simulink model "MANUFACTURINGCELL"  (R2026a)
settings: Solver=VariableStepAuto  StopTime=1000.0
undefined symbols (not defined in the file): m, n
libraries: sldelib x3
settings Model: Creator=Sayandip Mallick  LastModifiedBy=Nilesh Banik

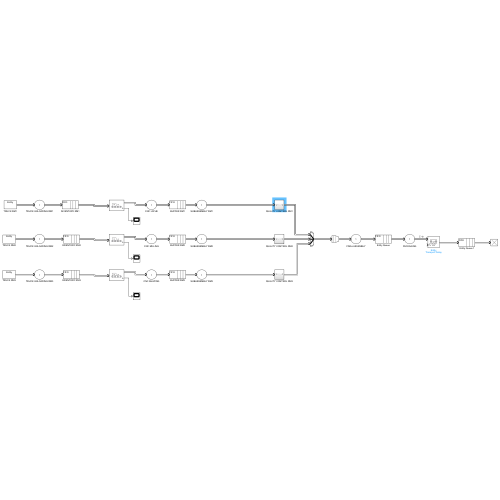
[thumbnail: Simulink's stored preview of the top-level diagram]
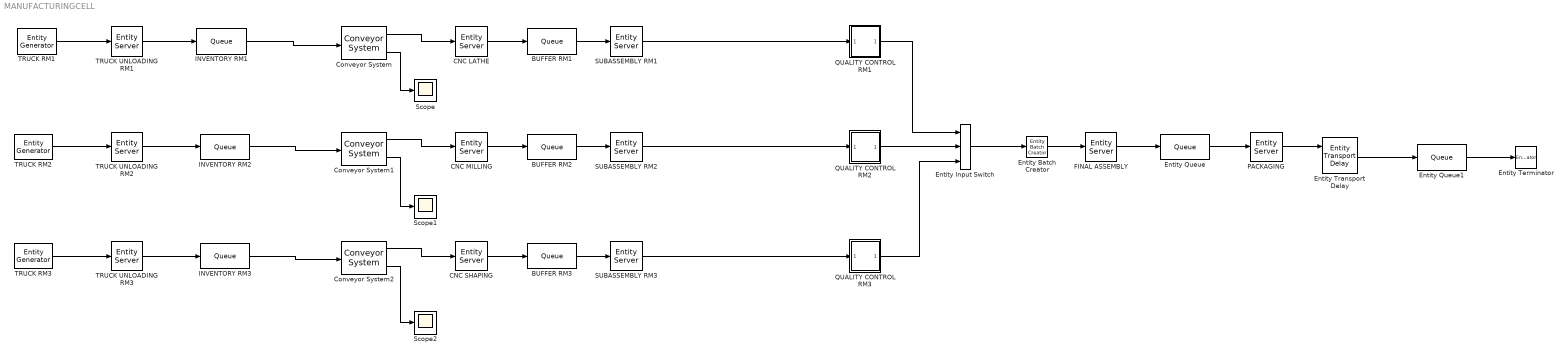
== system MANUFACTURINGCELL ==
  BUFFER RM1 : Queue  InputPortMessageModes=m  OutputPortMessageModes=m
  BUFFER RM2 : Queue  InputPortMessageModes=m  OutputPortMessageModes=m
  BUFFER RM3 : Queue  InputPortMessageModes=m  OutputPortMessageModes=m
  CNC LATHE : EntityServer  InputPortMessageModes=m  OutputPortMessageModes=m  Capacity=1
  CNC MILLING : EntityServer  InputPortMessageModes=m  OutputPortMessageModes=m  Capacity=1
  CNC SHAPING : EntityServer  InputPortMessageModes=m  OutputPortMessageModes=m  Capacity=1
  Conveyor System : sldelib/Conveyor System  mConveyorLength=10  mConveyorSpeedSource=Dialog  mConveyorSpeed=2  mInitialConveyorSpeed=1000  mMinDisBetEntity=1  mEntityLengthSource=Dialog  mEntityLength=1  mEntityLengthAttrName=Length  mOutputBlockedOpt=Pause  mErrorUponFullOpt=on  mNumEntitiesDepOpt=off  mNumEntitiesInBlockOpt=on  mEntityPendingOpt=off  mNumExtractedFromBlockOpt=off  mConveyorSpeedOpt=off
  Conveyor System1 : sldelib/Conveyor System  mConveyorLength=10  mConveyorSpeedSource=Dialog  mConveyorSpeed=2  mInitialConveyorSpeed=1000  mMinDisBetEntity=1  mEntityLengthSource=Dialog  mEntityLength=1  mEntityLengthAttrName=Length  mOutputBlockedOpt=Pause  mErrorUponFullOpt=on  mNumEntitiesDepOpt=off  mNumEntitiesInBlockOpt=on  mEntityPendingOpt=off  mNumExtractedFromBlockOpt=off  mConveyorSpeedOpt=off
  Conveyor System2 : sldelib/Conveyor System  mConveyorLength=10  mConveyorSpeedSource=Dialog  mConveyorSpeed=2  mInitialConveyorSpeed=1000  mMinDisBetEntity=1  mEntityLengthSource=Dialog  mEntityLength=1  mEntityLengthAttrName=Length  mOutputBlockedOpt=Pause  mErrorUponFullOpt=on  mNumEntitiesDepOpt=off  mNumEntitiesInBlockOpt=on  mEntityPendingOpt=off  mNumExtractedFromBlockOpt=off  mConveyorSpeedOpt=off
  Entity Input Switch : EntityInputSwitch  InputPortMessageModes=m,m,m  OutputPortMessageModes=m  NumberInputPorts=3
      settings: InputPortMap=u1,u2,u3
  Entity Transport Delay : EntityTransportDelay  InputPortMessageModes=m,n  OutputPortMessageModes=m
  Entity Batch Creator : EntityBatchCreator  InputPortMessageModes=m  OutputPortMessageModes=m  NumberOfEntitiesInBatch=3
      settings: OutputPortMap=o4
  Entity Queue : Queue  InputPortMessageModes=m  OutputPortMessageModes=m
  Entity Queue1 : Queue  InputPortMessageModes=m  OutputPortMessageModes=m
  Entity Terminator : EntityTerminator  InputPortMessageModes=m
  FINAL ASSEMBLY : EntityServer  InputPortMessageModes=m  OutputPortMessageModes=m  Capacity=1
  INVENTORY RM1 : Queue  InputPortMessageModes=m  OutputPortMessageModes=m
  INVENTORY RM2 : Queue  InputPortMessageModes=m  OutputPortMessageModes=m
  INVENTORY RM3 : Queue  InputPortMessageModes=m  OutputPortMessageModes=m
  PACKAGING : EntityServer  InputPortMessageModes=m  OutputPortMessageModes=m  Capacity=1
  QUALITY CONTROL RM1 : Subsystem
  QUALITY CONTROL RM2 : Subsystem
  QUALITY CONTROL RM3 : Subsystem
  SUBASSEMBLY RM1 : EntityServer  InputPortMessageModes=m  OutputPortMessageModes=m  Capacity=1
  SUBASSEMBLY RM2 : EntityServer  InputPortMessageModes=m  OutputPortMessageModes=m  Capacity=1
  SUBASSEMBLY RM3 : EntityServer  InputPortMessageModes=m  OutputPortMessageModes=m  Capacity=1
  Scope : Scope
      settings: ActiveDisplayYMinimum=-0.028729918999930576  ActiveDisplayYMaximum=0.73866164792601829
  Scope1 : Scope
  Scope2 : Scope
      settings: DataLoggingVariableName=ScopeData2
  TRUCK RM1 : EntityGenerator  OutputPortMessageModes=m  Period=300  EntityType=Structured  EntityTypeName=Entity
  TRUCK RM2 : EntityGenerator  OutputPortMessageModes=m  Period=300  EntityType=Structured  EntityTypeName=Entity
  TRUCK RM3 : EntityGenerator  OutputPortMessageModes=m  Period=300  EntityType=Structured  EntityTypeName=Entity
  TRUCK UNLOADING RM1 : EntityServer  InputPortMessageModes=m  OutputPortMessageModes=m  Capacity=1
  TRUCK UNLOADING RM2 : EntityServer  InputPortMessageModes=m  OutputPortMessageModes=m  Capacity=1
  TRUCK UNLOADING RM3 : EntityServer  InputPortMessageModes=m  OutputPortMessageModes=m  Capacity=1
  wires:
  TRUCK RM1/1 -> TRUCK UNLOADING RM1/1
  TRUCK UNLOADING RM1/1 -> INVENTORY RM1/1
  INVENTORY RM1/1 -> Conveyor System/1
  TRUCK UNLOADING RM2/1 -> INVENTORY RM2/1
  TRUCK RM2/1 -> TRUCK UNLOADING RM2/1
  TRUCK UNLOADING RM3/1 -> INVENTORY RM3/1
  TRUCK RM3/1 -> TRUCK UNLOADING RM3/1
  CNC LATHE/1 -> BUFFER RM1/1
  CNC MILLING/1 -> BUFFER RM2/1
  CNC SHAPING/1 -> BUFFER RM3/1
  BUFFER RM1/1 -> SUBASSEMBLY RM1/1
  BUFFER RM2/1 -> SUBASSEMBLY RM2/1
  BUFFER RM3/1 -> SUBASSEMBLY RM3/1
  SUBASSEMBLY RM1/1 -> QUALITY CONTROL RM1/1(In1)
  SUBASSEMBLY RM2/1 -> QUALITY CONTROL RM2/1(In1)
  SUBASSEMBLY RM3/1 -> QUALITY CONTROL RM3/1(In1)
  QUALITY CONTROL RM1/1(Out1) -> Entity Input Switch/1
  QUALITY CONTROL RM2/1(Out1) -> Entity Input Switch/2
  QUALITY CONTROL RM3/1(Out1) -> Entity Input Switch/3
  Entity Input Switch/1 -> Entity Batch Creator/1
  Entity Batch Creator/1 -> FINAL ASSEMBLY/1
  FINAL ASSEMBLY/1 -> Entity Queue/1
  Entity Queue/1 -> PACKAGING/1
  PACKAGING/1 -> Entity Transport Delay/1
  Entity Transport Delay/1 -> Entity Queue1/1
  Entity Queue1/1 -> Entity Terminator/1
  Conveyor System/1 -> CNC LATHE/1
  INVENTORY RM2/1 -> Conveyor System1/1
  Conveyor System1/1 -> CNC MILLING/1
  Conveyor System2/1 -> CNC SHAPING/1
  INVENTORY RM3/1 -> Conveyor System2/1
  Conveyor System/2 -> Scope/1
  Conveyor System1/2 -> Scope1/1
  Conveyor System2/2 -> Scope2/1

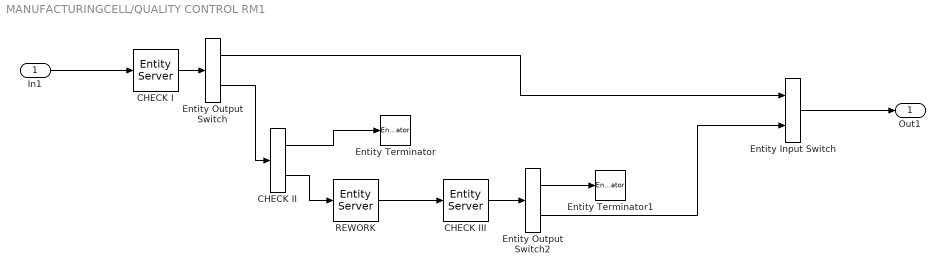
== system MANUFACTURINGCELL/QUALITY CONTROL RM1 ==
  In1 : Inport
  CHECK I : EntityServer  InputPortMessageModes=m  OutputPortMessageModes=m  Capacity=1
  CHECK II : EntityOutputSwitch  InputPortMessageModes=m  OutputPortMessageModes=m,m  SwitchAttributeName=Attribute1
  CHECK III : EntityServer  InputPortMessageModes=m  OutputPortMessageModes=m  Capacity=1
  Entity Input Switch : EntityInputSwitch  InputPortMessageModes=m,m  OutputPortMessageModes=m
  Entity Output Switch : EntityOutputSwitch  InputPortMessageModes=m  OutputPortMessageModes=m,m  SwitchingCriterion=From attribute  SwitchAttributeName=Attribute1
  Entity Output Switch2 : EntityOutputSwitch  InputPortMessageModes=m  OutputPortMessageModes=m,m  SwitchAttributeName=Attribute1
  Entity Terminator : EntityTerminator  InputPortMessageModes=m
  Entity Terminator1 : EntityTerminator  InputPortMessageModes=m
  REWORK : EntityServer  InputPortMessageModes=m  OutputPortMessageModes=m  Capacity=1
  Out1 : Outport
  wires:
  Entity Output Switch/2 -> CHECK II/1
  CHECK II/2 -> REWORK/1
  CHECK III/1 -> Entity Output Switch2/1
  Entity Output Switch2/1 -> Entity Terminator1/1
  CHECK I/1 -> Entity Output Switch/1
  REWORK/1 -> CHECK III/1
  CHECK II/1 -> Entity Terminator/1
  In1/1 -> CHECK I/1
  Entity Output Switch/1 -> Entity Input Switch/1
  Entity Output Switch2/2 -> Entity Input Switch/2
  Entity Input Switch/1 -> Out1/1

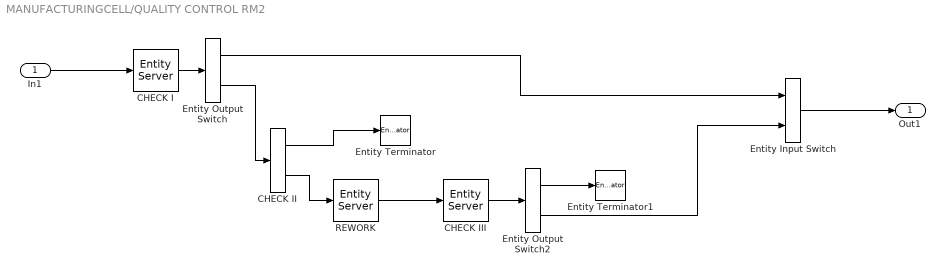
== system MANUFACTURINGCELL/QUALITY CONTROL RM2 ==
  In1 : Inport
  CHECK I : EntityServer  InputPortMessageModes=m  OutputPortMessageModes=m  Capacity=1
  CHECK II : EntityOutputSwitch  InputPortMessageModes=m  OutputPortMessageModes=m,m  SwitchAttributeName=Attribute1
  CHECK III : EntityServer  InputPortMessageModes=m  OutputPortMessageModes=m  Capacity=1
  Entity Input Switch : EntityInputSwitch  InputPortMessageModes=m,m  OutputPortMessageModes=m
  Entity Output Switch : EntityOutputSwitch  InputPortMessageModes=m  OutputPortMessageModes=m,m  SwitchingCriterion=From attribute  SwitchAttributeName=Attribute1
  Entity Output Switch2 : EntityOutputSwitch  InputPortMessageModes=m  OutputPortMessageModes=m,m  SwitchAttributeName=Attribute1
  Entity Terminator : EntityTerminator  InputPortMessageModes=m
  Entity Terminator1 : EntityTerminator  InputPortMessageModes=m
  REWORK : EntityServer  InputPortMessageModes=m  OutputPortMessageModes=m  Capacity=1
  Out1 : Outport
  wires:
  Entity Output Switch/2 -> CHECK II/1
  CHECK II/2 -> REWORK/1
  CHECK III/1 -> Entity Output Switch2/1
  Entity Output Switch2/1 -> Entity Terminator1/1
  CHECK I/1 -> Entity Output Switch/1
  REWORK/1 -> CHECK III/1
  CHECK II/1 -> Entity Terminator/1
  In1/1 -> CHECK I/1
  Entity Output Switch/1 -> Entity Input Switch/1
  Entity Output Switch2/2 -> Entity Input Switch/2
  Entity Input Switch/1 -> Out1/1

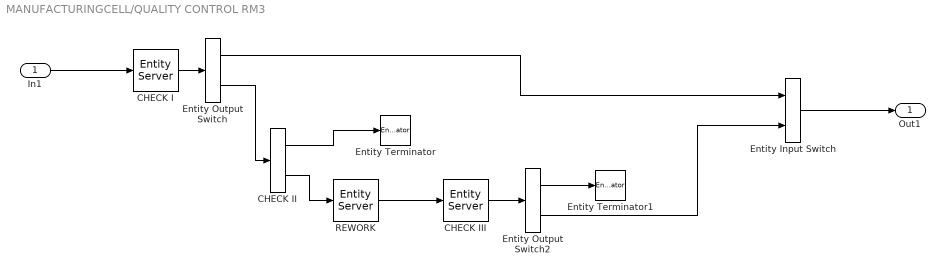
== system MANUFACTURINGCELL/QUALITY CONTROL RM3 ==
  In1 : Inport
  CHECK I : EntityServer  InputPortMessageModes=m  OutputPortMessageModes=m  Capacity=1
  CHECK II : EntityOutputSwitch  InputPortMessageModes=m  OutputPortMessageModes=m,m  SwitchAttributeName=Attribute1
  CHECK III : EntityServer  InputPortMessageModes=m  OutputPortMessageModes=m  Capacity=1
  Entity Input Switch : EntityInputSwitch  InputPortMessageModes=m,m  OutputPortMessageModes=m
  Entity Output Switch : EntityOutputSwitch  InputPortMessageModes=m  OutputPortMessageModes=m,m  SwitchingCriterion=From attribute  SwitchAttributeName=Attribute1
  Entity Output Switch2 : EntityOutputSwitch  InputPortMessageModes=m  OutputPortMessageModes=m,m  SwitchAttributeName=Attribute1
  Entity Terminator : EntityTerminator  InputPortMessageModes=m
  Entity Terminator1 : EntityTerminator  InputPortMessageModes=m
  REWORK : EntityServer  InputPortMessageModes=m  OutputPortMessageModes=m  Capacity=1
  Out1 : Outport
  wires:
  Entity Output Switch/2 -> CHECK II/1
  CHECK II/2 -> REWORK/1
  CHECK III/1 -> Entity Output Switch2/1
  Entity Output Switch2/1 -> Entity Terminator1/1
  CHECK I/1 -> Entity Output Switch/1
  REWORK/1 -> CHECK III/1
  CHECK II/1 -> Entity Terminator/1
  In1/1 -> CHECK I/1
  Entity Output Switch/1 -> Entity Input Switch/1
  Entity Output Switch2/2 -> Entity Input Switch/2
  Entity Input Switch/1 -> Out1/1
